simulink library "sm_linear_actuator_lib"  (R2021b)
settings: Solver=ode45  StartTime=0.0  StopTime=10.0  RelTol=1e-3  EnableMultiTasking=on
undefined symbols (not defined in the file or in its folder): X, Y, Z
libraries: sm_lib x28, $bdroot x7
settings Model: Creator=The MathWorks, Inc.  LastModifiedBy=The MathWorks, Inc.
settings SolverCC: AlgebraicLoopSolver=TrustRegion
settings DataIOCC: LimitDataPoints=on  SaveFormat=Array  ReturnWorkspaceOutputs=off
settings OptimizationCC: LifeSpan=inf
settings DebuggingCC: SolverPrmCheckMsg=warning  AllowSymbolicDim=off  SFUnexpectedBacktrackingDiag=warning  SFNoUnconditionalDefaultTransitionDiag=warning  SFExecutionAtInitializationDiag=none  SFMachineParentedDataDiag=warning  ArithmeticOperatorsInVariantConditions=warning
settings HardwareCC: ProdBitPerPointer=32  ProdBitPerSizeT=32  ProdBitPerPtrDiffT=32  ProdLargestAtomicFloat=None  ProdIntDivRoundTo=Undefined  ProdEndianess=Unspecified  ProdWordSize=32  ProdHWDeviceType=32-bit Generic
settings ModelReferenceCC: PropagateSignalLabelsOutOfModel=off
settings SFSimCC: SimUseLocalCustomCode=off  CustomCodeUndefinedFunction=UseInterfaceOnly
settings RTWCC: RTWUseLocalCustomCode=off
settings CodeAppCC: StateflowObjectComments=on
settings GRTTargetCC: TargetLangStandard=C89/C90 (ANSI)
settings ConfigComp: CovMetricSettings=dw  CovSaveCumulativeToWorkspaceVar=on  CovSaveSingleToWorkspaceVar=on  CovExternalEMLEnable=off  CovSFcnEnable=off

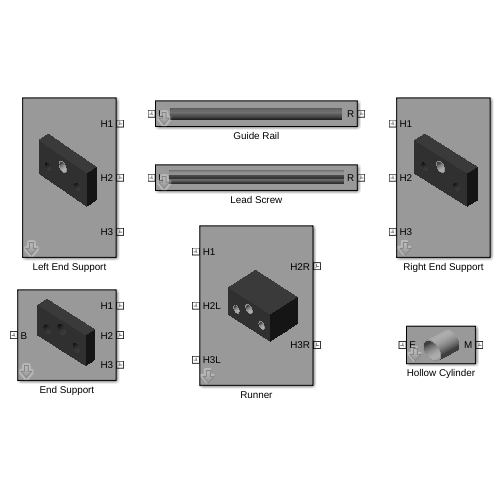
[thumbnail: Simulink's stored preview of the top-level diagram]
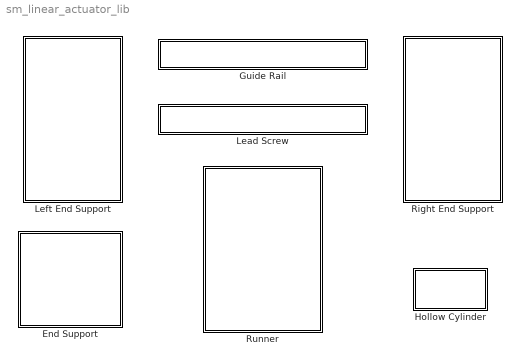
== system sm_linear_actuator_lib ==
  End Support : Subsystem  StatePerturbationForJacobian=1.0e-05  mask(End Support){H=50, W=100, D=20, R1=8.5, R2=7.5, hole1_offset=[0 35], hole2_offset=[30 20], hole3_offset=[-30 20], rho=7800, color=[0.3 0.3 0.3]}
      mask prompts: H "Height (mm)"; W "Width (mm)"; D "Depth (mm)"; R1 "Hole 1 Radius (mm)"; R2 "Holes 2 and 3 Radii (mm)"; hole1_offset "Hole 1 Offset [x y] (mm)"; hole2_offset "Hole 2 Offset [x y] (mm)"; hole3_offset "Hole 3 Offset [x y] (mm)"; rho "Density (kg/m^3)"; color "Color [r g b]"
      mask help:
      | This block models the base part of the end supports for the linear actuator.
      |
      | Port B corresponds to the center of the bottom face of the element.
      |
      | Ports H1, H2 and H3 correspond to the central point of each hole respectively.
      |
      | Each port is located at the midsection of the element.
      mask init:
      | hole_points = 40;
      | 
      | qHole1 = linspace(pi/2, pi/2-2*pi, hole_points);
      | hole1 = [R1*cos(qHole1);
      |          R1*sin(qHole1)+hole1_offset(2)]';
      | 
      | qHole2 = linspace(0, -2*pi, hole_points);
      | hole2 = [R2*cos(qHole2)+hole2_offset(1); 
      |          R2*sin(qHole2)+hole2_offset(2)]';
      | 
      | qHole3 = linspace(pi, -pi, hole_points);
      | hole3 = [R2*cos(qHole3)+hole3_offset(1); 
      |          R2*sin(qHole3)+hole3_offset(2)]';
      | 
      | extrusion_points = [ 0     0;
      |                      0.5*W 0;
      |                      0.5*W hole2_offset(2);
      |                      hole2;
      |                      0.5*W hole2_offset(2);
      |                      0.5*W H;
      |                      0     H;
      |                      hole1;
      |                      0     H;
      |                     -0.5*W H;
      |                     -0.5*W hole3_offset(2);
      |                      hole3;
      |                     -0.5*W hole3_offset(2);
      |                     -0.5*W 0];
      mask DialogControl Container4 Prompt: Dimensions
      mask DialogControl Container9 Prompt: Material Properties
      mask Display:
      | image(fullfile(matlabroot,'toolbox','physmod','sm','smdemos','linear_actuator','images','sm_linear_actuator_end_support.png'));
      | port_label('lconn',1,'B');
      | port_label('rconn',1,'H1');
      | port_label('rconn',2,'H2');
      | port_label('rconn',3,'H3');
  Guide Rail : Subsystem  StatePerturbationForJacobian=1.0e-05  mask(Guide Rail){L=500, R=6, rho=7800, color=[0.5 0.5 0.5]}
      mask prompts: L "Length (mm)"; R "Radius (mm)"; rho "Density (kg/m^3)"; color "Color [r g b]"
      mask help:
      | This block models a guide rail of the linear actuator.
      |
      | The ports L and R correspond to the central points of the two end faces.
      mask DialogControl Container4 Prompt: Dimensions
      mask DialogControl Container5 Prompt: Material Properties
      mask Display:
      | image(fullfile(matlabroot,'toolbox','physmod','sm','smdemos','linear_actuator','images','sm_linear_actuator_guide_rail.png'));
      | port_label('lconn',1,'L');
      | port_label('rconn',1,'R');
  Hollow Cylinder : Subsystem  StatePerturbationForJacobian=1.0e-05  mask(Hollow Cylinder){R=10, T=1, L=20, rho=7800, color=[0.9 0.9 0.9]}
      mask prompts: R "Outer Radius (mm)"; T "Thickness (mm)"; L "Length (mm)"; rho "Density (kg/m^3)"; color "Color [r g b]"
      mask help:
      | This block models a hollow cylinder element.
      |
      | The port E corresponds to the center of the cross-section at the left end.
      |
      | The port M corresponds to the center of the cross-section at the midpoint of the element.
      mask init:
      | iR = R - T;
      | 
      | revolution_points = [iR  L/2;
      |                      iR -L/2;
      |                      R  -L/2;
      |                      R   L/2];
      mask DialogControl Tab01 Prompt: Dimensions
      mask DialogControl Tab02 Prompt: Material Properties
      mask Display:
      | image(fullfile(matlabroot,'toolbox','physmod','sm','smdemos','linear_actuator','images','sm_linear_actuator_hollow_cylinder.png'));
      | port_label('lconn',1,'E');
      | port_label('rconn',1,'M');
  Lead Screw : Subsystem  StatePerturbationForJacobian=1.0e-05  mask(Lead Screw){L=500, R=6, rho=7800, iColor=[0.3 0.3 0.3], oColor=[0.7 0.7 0.7]}
      mask prompts: L "Length (mm)"; R "Radius (mm)"; rho "Density (kg/m^3)"; iColor "Inner Color [r g b]"; oColor "Outer Color [r g b]"
      mask help:
      | This block models the lead screw of the linear actuator.
      |
      | Ports L and R correspond to the central points of the two end faces.
      mask init:
      | x = 0.25*R;
      | 
      | theta = acos(x / R);
      | 
      | theta_arc = pi - 2 * theta;
      | 
      | theta_top_arc = linspace(theta, theta + theta_arc, 20);
      | theta_left_arc = linspace(theta + theta_arc, theta + pi, 20);
      | theta_bottom_arc = linspace(theta + pi, theta + pi + theta_arc, 20);
      | theta_right_arc = linspace(theta + pi + theta_arc, theta + 2*pi, 20);
      | 
      | left_section = [R*cos(theta_left_arc);
      |                   R*sin(theta_left_arc)]';
      | 
      | middle_section = [R*cos(theta_top_arc) R*cos(theta_bottom_arc);
      |                   R*sin(theta_top_arc) R*sin(theta_bottom_arc)]';
      | 
      | right_section = [R*cos(theta_right_arc);
      |                   R*sin(theta_right_arc)]';
      mask DialogControl Container4 Prompt: Dimensions
      mask DialogControl Container5 Prompt: Material Properties
      mask Display:
      | image(fullfile(matlabroot,'toolbox','physmod','sm','smdemos','linear_actuator','images','sm_linear_actuator_lead_screw.png'));
      | port_label('lconn',1,'L');
      | port_label('rconn',1,'R');
  Left End Support : Subsystem  StatePerturbationForJacobian=1.0e-05  mask(Left End Support){H=50, W=100, D=20, R1=7, R2=6, T=1.5, hole1_offset=[0 35], hole2_offset=[30 20], hole3_offset=[-30 20], rho=7800, sColor=[0.3 0.3 0.3], bColor=[0.9 0.9 0.9]}
      mask prompts: H "Height (mm)"; W "Width (mm)"; D "Depth (mm)"; R1 "Hole 1 Radius (mm)"; R2 "Holes 2 and 3 Radii (mm)"; T "Bearing Thickness (mm)"; hole1_offset "Hole 1 Offset [x y] (mm)"; hole2_offset "Hole 2 Offset [x y] (mm)"; hole3_offset "Hole 3 Offset [x y] (mm)"; rho "Density (mg/m^3)"; sColor "Support Color [r g b]"; bColor "Bearing Color [r g b]"
      mask help:
      | This block models the left end support of the linear actuator. The block comprises one End Support and one Hollow Cylinder which models the bearing on which the lead screw rotates.
      |
      | Ports H1, H2 and H3 correspond to the center point of each hole. Each is located on the rear face of the element.
      mask DialogControl Container4 Prompt: Dimensions
      mask DialogControl Container5 Prompt: Material Properties
      mask Display:
      | image(fullfile(matlabroot,'toolbox','physmod','sm','smdemos','linear_actuator','images','sm_linear_actuator_left_end_support.png'));
      | port_label('rconn',1,'H1');
      | port_label('rconn',2,'H2');
      | port_label('rconn',3,'H3');
  Right End Support : Subsystem  StatePerturbationForJacobian=1.0e-05  mask{H=50, W=100, D=20, R1=7, R2=6, T=1.5, hole1_offset=[0 35], hole2_offset=[30 20], hole3_offset=[-30 20], rho=7800, sColor=[0.3 0.3 0.3], bColor=[0.9 0.9 0.9]}
      mask prompts: H "Height (mm)"; W "Width (mm)"; D "Depth (mm)"; R1 "Hole 1 Radius (mm)"; R2 "Holes 2 and 3 Radii (mm)"; T "Bearing Thickness (mm)"; hole1_offset "Hole 1 Offset [x y] (mm)"; hole2_offset "Hole 2 Offset [x y] (mm)"; hole3_offset "Hole 3 Offset [x y] (mm)"; rho "Density (mg/m^3)"; sColor "Support Color [r g b]"; bColor "Bearing Color [r g b]"
      mask help:
      | This block models the right end support of the linear actuator. The block comprises one End Support and one Hollow Cylinder which models the bearing on which the lead screw rotates.
      |
      | Ports H1, H2 and H3 correspond to the center point of each hole. Each is located on the rear face of the element.
      mask DialogControl Container4 Prompt: Dimensions
      mask DialogControl Container5 Prompt: Material Properties
      mask Display:
      | image(fullfile(matlabroot,'toolbox','physmod','sm','smdemos','linear_actuator','images','sm_linear_actuator_right_end_support.png'));
      | port_label('lconn',1,'H1');
      | port_label('lconn',2,'H2');
      | port_label('lconn',3,'H3');
  Runner : Subsystem  StatePerturbationForJacobian=1.0e-05  mask(Runner){H=50, W=100, D=65, R1=7, R2=6, T=1.5, hole1_offset=[0 35], hole2_offset=[30 20], hole3_offset=[-30 20], rho=7800, rColor=[0.3 0.3 0.3], bColor=[0.9 0.9 0.9]}
      mask prompts: H "Height (mm)"; W "Width (mm)"; D "Depth (mm)"; R1 "Hole 1 Radius (mm)"; R2 "Holes 2 and 3 Radii (mm)"; T "Bearing Thickness"; hole1_offset "Hole 1 Offset [x y] (mm)"; hole2_offset "Hole 2 Offset [x y] (mm)"; hole3_offset "Hole 3 Offset [x y] (mm)"; rho "Density (kg/m^3)"; rColor "Runner Color [r g b]"; bColor "Bearing Color [r g b]"
      mask help:
      | This block models the runner of the linear actuator. The block contains three Hollow Cylinder elements which model the bearings on which the runner slides and connect the runner to the lead screw.
      |
      | Port H1 corresponds to the lead screw connection and is located at the central point of hole 1.
      |
      | Ports H2L, H3L, H2R and H3R correspond to the connection points to the guide rails and are located at the center points of the holes on the front and rear faces.
      mask init:
      | hole_points = 40;
      | 
      | qHole1 = linspace(pi/2, pi/2-2*pi, hole_points);
      | r1 = R1+T;
      | hole1 = [r1*cos(qHole1);
      |          r1*sin(qHole1)+hole1_offset(2)]';
      | 
      | qHole2 = linspace(0, -2*pi, hole_points);
      | r2 = R2+T;
      | hole2 = [r2*cos(qHole2)+hole2_offset(1); 
      |          r2*sin(qHole2)+hole2_offset(2)]';
      | 
      | qHole3 = linspace(pi, -pi, hole_points);
      | hole3 = [r2*cos(qHole3)+hole3_offset(1); 
      |          r2*sin(qHole3)+hole3_offset(2)]';
      | 
      | extrusion_points = [ 0     0;
      |                      0.5*W 0;
      |                      0.5*W hole2_offset(2);
      |                      hole2;
      |                      0.5*W hole2_offset(2);
      |                      0.5*W H;
      |                      0     H;
      |                      hole1;
      |                      0     H;
      |                     -0.5*W H;
      |                     -0.5*W hole3_offset(2);
      |                      hole3;
      |                     -0.5*W hole3_offset(2);
      |                     -0.5*W 0];
      mask DialogControl Container4 Prompt: Runner Dimensions
      mask DialogControl Container9 Prompt: Material Properties
      mask Display:
      | image(fullfile(matlabroot,'toolbox','physmod','sm','smdemos','linear_actuator','images','sm_linear_actuator_runner.png'));
      | port_label('lconn',1,'H1');
      | port_label('lconn',2,'H2L');
      | port_label('lconn',3,'H3L');
      | port_label('rconn',1,'H2R');
      | port_label('rconn',2,'H3R');

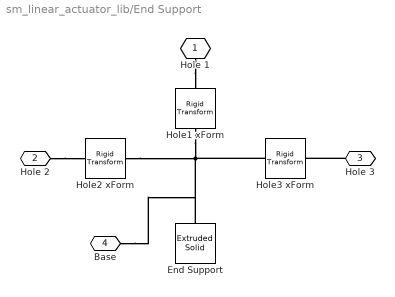
== system sm_linear_actuator_lib/End Support ==
  End Support : sm_lib/Body Elements/Extruded Solid  StatePerturbationForJacobian=1.0e-05  GraphicAmbientColor=[0.15 0.15 0.15 1.0]  BasedOnType=Density  CenterOfMass=[0 0 0]  CenterOfMassUnits=m  GraphicDiffuseColor=color  ExportConvexHullGeometry=off  ExtrusionCrossSection=extrusion_points  ExtrusionCrossSectionUnits=mm  Density=rho  DensityUnits=kg/(m^3)  DoExposeReferenceFrame=on  GraphicEmissiveColor=[0.0 0.0 0.0 1.0]  ExportEntireGeometry=off  ExtrusionLength=D  ExtrusionLengthUnits=mm  ExtrusionType=General  SerializedFrames=<Frames/>  MarkerShape=Sphere  MarkerSize=10  GraphicType=FromGeometry  InertiaType=CalculateFromGeometry  Mass=1  MassUnits=kg  MomentsOfInertia=[1 1 1]  MomentsOfInertiaUnits=kg*m^2  PolygonNumSides=3  GraphicOpacity=1.0  PolygonOuterRadius=1  PolygonOuterRadiusUnits=m  ProductsOfInertia=[0 0 0]  ProductsOfInertiaUnits=kg*m^2  GraphicShininess=75  GraphicSpecularColor=[0.5 0.5 0.5 1.0]  GraphicVisPropType=SimpleVisualProperties
  Hole1 xForm : sm_lib/Frames and Transforms/Rigid Transform  StatePerturbationForJacobian=1.0e-05  TranslationMethod=Cartesian  TranslationStandardOffset=0  TranslationLengthUnit=mm  TranslationStandardAxis=+Z  TranslationCartesianOffset=[hole1_offset 0]  TranslationROffset=0  TranslationROffsetUnits=m  TranslationZOffset=0  TranslationZOffsetUnits=m  TranslationThetaOffset=0  TranslationThetaOffsetUnits=deg  RotationMethod=None  RotationAngleUnits=deg  RotationStandardAxis=+Z  RotationAngle=0.0  RotationArbitraryAxis=[0 0 1]  FollAlignAxisA=+X  BaseAlignAxisA=+Y  FollAlignAxisB=+Y  BaseAlignAxisB=+Z  RotationSequenceAxes=FollowerAxes  RotationSequence=XYX  RotationSequenceAngles=[0 0 0]  RotationSequenceAnglesUnits=deg  RotationMatrix=[1 0 0; 0 1 0; 0 0 1]
  Hole2 xForm : sm_lib/Frames and Transforms/Rigid Transform  StatePerturbationForJacobian=1.0e-05  TranslationMethod=Cartesian  TranslationStandardOffset=0  TranslationLengthUnit=mm  TranslationStandardAxis=+Z  TranslationCartesianOffset=[hole2_offset 0]  TranslationROffset=0  TranslationROffsetUnits=m  TranslationZOffset=0  TranslationZOffsetUnits=m  TranslationThetaOffset=0  TranslationThetaOffsetUnits=deg  RotationMethod=None  RotationAngleUnits=deg  RotationStandardAxis=+Z  RotationAngle=0.0  RotationArbitraryAxis=[0 0 1]  FollAlignAxisA=+X  BaseAlignAxisA=+Y  FollAlignAxisB=+Y  BaseAlignAxisB=+Z  RotationSequenceAxes=FollowerAxes  RotationSequence=XYX  RotationSequenceAngles=[0 0 0]  RotationSequenceAnglesUnits=deg  RotationMatrix=[1 0 0; 0 1 0; 0 0 1]
  Hole3 xForm : sm_lib/Frames and Transforms/Rigid Transform  StatePerturbationForJacobian=1.0e-05  TranslationMethod=Cartesian  TranslationStandardOffset=0  TranslationLengthUnit=mm  TranslationStandardAxis=+Z  TranslationCartesianOffset=[hole3_offset 0]  TranslationROffset=0  TranslationROffsetUnits=m  TranslationZOffset=0  TranslationZOffsetUnits=m  TranslationThetaOffset=0  TranslationThetaOffsetUnits=deg  RotationMethod=None  RotationAngleUnits=deg  RotationStandardAxis=+Z  RotationAngle=0.0  RotationArbitraryAxis=[0 0 1]  FollAlignAxisA=+X  BaseAlignAxisA=+Y  FollAlignAxisB=+Y  BaseAlignAxisB=+Z  RotationSequenceAxes=FollowerAxes  RotationSequence=XYX  RotationSequenceAngles=[0 0 0]  RotationSequenceAnglesUnits=deg  RotationMatrix=[1 0 0; 0 1 0; 0 0 1]
  Hole 1 : PMIOPort  StatePerturbationForJacobian=1.0e-05  Side=Right
  Hole 2 : PMIOPort  StatePerturbationForJacobian=1.0e-05  Port=2  Side=Right
  Hole 3 : PMIOPort  StatePerturbationForJacobian=1.0e-05  Port=3  Side=Right
  Base : PMIOPort  StatePerturbationForJacobian=1.0e-05  Port=4  Side=Left
  connections:
  Hole 3/RConn1 -- Hole3 xForm/RConn1
  Hole 2/RConn1 -- Hole2 xForm/RConn1
  Hole 1/RConn1 -- Hole1 xForm/RConn1
  Hole3 xForm/LConn1 -- Base/RConn1 -- End Support/RConn1 -- Hole2 xForm/LConn1 -- Hole1 xForm/LConn1

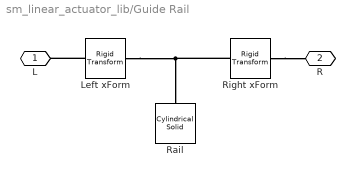
== system sm_linear_actuator_lib/Guide Rail ==
  Left xForm : sm_lib/Frames and Transforms/Rigid Transform  StatePerturbationForJacobian=1.0e-05  TranslationMethod=StandardAxis  TranslationStandardOffset=L/2  TranslationLengthUnit=mm  TranslationStandardAxis=+Z  TranslationCartesianOffset=[0 0 0]  TranslationROffset=0  TranslationROffsetUnits=m  TranslationZOffset=0  TranslationZOffsetUnits=m  TranslationThetaOffset=0  TranslationThetaOffsetUnits=deg  RotationMethod=AlignedAxes  RotationAngleUnits=deg  RotationStandardAxis=+Z  RotationAngle=0.0  RotationArbitraryAxis=[0 0 1]  FollAlignAxisA=+Z  BaseAlignAxisA=-Z  FollAlignAxisB=+Y  BaseAlignAxisB=+Y  RotationSequenceAxes=FollowerAxes  RotationSequence=XYX  RotationSequenceAngles=[0 0 0]  RotationSequenceAnglesUnits=deg  RotationMatrix=[1 0 0; 0 1 0; 0 0 1]
  Rail : sm_lib/Body Elements/Cylindrical Solid  StatePerturbationForJacobian=1.0e-05  GraphicAmbientColor=[0.15 0.15 0.15 1.0]  BasedOnType=Density  CenterOfMass=[0 0 0]  CenterOfMassUnits=m  GraphicDiffuseColor=color  CylinderLength=L  CylinderLengthUnits=mm  CylinderRadius=R  CylinderRadiusUnits=mm  Density=rho  DensityUnits=kg/(m^3)  DoExposeReferenceFrame=on  GraphicEmissiveColor=[0.0 0.0 0.0 1.0]  ExportEntireGeometry=off  SerializedFrames=<Frames/>  MarkerShape=Sphere  MarkerSize=10  GraphicType=FromGeometry  InertiaType=CalculateFromGeometry  Mass=1  MassUnits=kg  MomentsOfInertia=[1 1 1]  MomentsOfInertiaUnits=kg*m^2  GraphicOpacity=1.0  ProductsOfInertia=[0 0 0]  ProductsOfInertiaUnits=kg*m^2  GraphicShininess=75  GraphicSpecularColor=[0.5 0.5 0.5 1.0]  GraphicVisPropType=SimpleVisualProperties
  Right xForm : sm_lib/Frames and Transforms/Rigid Transform  StatePerturbationForJacobian=1.0e-05  TranslationMethod=StandardAxis  TranslationStandardOffset=L/2  TranslationLengthUnit=mm  TranslationStandardAxis=-Z  TranslationCartesianOffset=[0 0 0]  TranslationROffset=0  TranslationROffsetUnits=m  TranslationZOffset=0  TranslationZOffsetUnits=m  TranslationThetaOffset=0  TranslationThetaOffsetUnits=deg  RotationMethod=None  RotationAngleUnits=deg  RotationStandardAxis=+Z  RotationAngle=0.0  RotationArbitraryAxis=[0 0 1]  FollAlignAxisA=+Z  BaseAlignAxisA=+Z  FollAlignAxisB=+Y  BaseAlignAxisB=+Y  RotationSequenceAxes=FollowerAxes  RotationSequence=XYX  RotationSequenceAngles=[0 0 0]  RotationSequenceAnglesUnits=deg  RotationMatrix=[1 0 0; 0 1 0; 0 0 1]
  L : PMIOPort  StatePerturbationForJacobian=1.0e-05  Side=Left
  R : PMIOPort  StatePerturbationForJacobian=1.0e-05  Port=2  Side=Right
  connections:
  Left xForm/RConn1 -- L/RConn1
  Right xForm/RConn1 -- R/RConn1
  Left xForm/LConn1 -- Rail/RConn1 -- Right xForm/LConn1

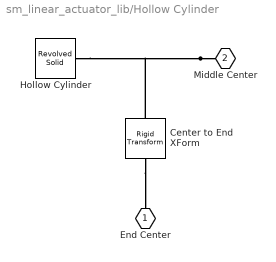
== system sm_linear_actuator_lib/Hollow Cylinder ==
  Center to End XForm : sm_lib/Frames and Transforms/Rigid Transform  StatePerturbationForJacobian=1.0e-05  TranslationMethod=StandardAxis  TranslationStandardOffset=L/2  TranslationLengthUnit=mm  TranslationStandardAxis=-Z  TranslationCartesianOffset=[0 0 0]  TranslationROffset=0  TranslationROffsetUnits=m  TranslationZOffset=0  TranslationZOffsetUnits=m  TranslationThetaOffset=0  TranslationThetaOffsetUnits=deg  RotationMethod=None  RotationAngleUnits=deg  RotationStandardAxis=+Z  RotationAngle=0  RotationArbitraryAxis=[0 0 1]  FollAlignAxisA=+X  BaseAlignAxisA=+Y  FollAlignAxisB=+Y  BaseAlignAxisB=+Z  RotationSequenceAxes=FollowerAxes  RotationSequence=XYX  RotationSequenceAngles=[0 0 0]  RotationSequenceAnglesUnits=deg  RotationMatrix=[1 0 0; 0 1 0; 0 0 1]
  Hollow Cylinder : sm_lib/Body Elements/Revolved Solid  StatePerturbationForJacobian=1.0e-05  GraphicAmbientColor=[0.15 0.15 0.15 1.0]  BasedOnType=Density  CenterOfMass=[0 0 0]  CenterOfMassUnits=m  GraphicDiffuseColor=color  ExportConvexHullGeometry=off  Density=rho  DensityUnits=kg/(m^3)  DoExposeReferenceFrame=on  GraphicEmissiveColor=[0.0 0.0 0.0 1.0]  ExportEntireGeometry=off  SerializedFrames=<Frames/>  MarkerShape=Sphere  MarkerSize=10  GraphicType=FromGeometry  InertiaType=CalculateFromGeometry  Mass=1  MassUnits=kg  MomentsOfInertia=[1 1 1]  MomentsOfInertiaUnits=kg*m^2  GraphicOpacity=1.0  ProductsOfInertia=[0 0 0]  ProductsOfInertiaUnits=kg*m^2  RevolutionCrossSection=revolution_points  RevolutionCrossSectionUnits=mm  RevolutionAngle=180  RevolutionAngleUnits=deg  RevolutionExtent=Full  GraphicShininess=75  GraphicSpecularColor=[0.5 0.5 0.5 1.0]  GraphicVisPropType=SimpleVisualProperties
  End Center : PMIOPort  StatePerturbationForJacobian=1.0e-05  Side=Left
  Middle Center : PMIOPort  StatePerturbationForJacobian=1.0e-05  Port=2  Side=Right
  connections:
  Center to End XForm/RConn1 -- End Center/RConn1
  Middle Center/RConn1 -- Center to End XForm/LConn1 -- Hollow Cylinder/RConn1

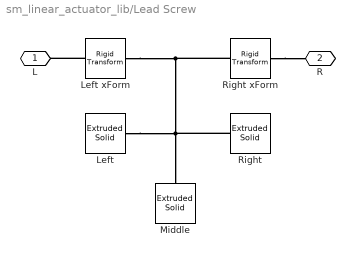
== system sm_linear_actuator_lib/Lead Screw ==
  Left : sm_lib/Body Elements/Extruded Solid  StatePerturbationForJacobian=1.0e-05  GraphicAmbientColor=[0.15 0.15 0.15 1.0]  BasedOnType=Density  CenterOfMass=[0 0 0]  CenterOfMassUnits=m  GraphicDiffuseColor=oColor  ExportConvexHullGeometry=off  ExtrusionCrossSection=left_section  ExtrusionCrossSectionUnits=mm  Density=rho  DensityUnits=kg/(m^3)  DoExposeReferenceFrame=on  GraphicEmissiveColor=[0.0 0.0 0.0 1.0]  ExportEntireGeometry=off  ExtrusionLength=L  ExtrusionLengthUnits=mm  ExtrusionType=General  SerializedFrames=<Frames/>  MarkerShape=Sphere  MarkerSize=10  GraphicType=FromGeometry  InertiaType=CalculateFromGeometry  Mass=1  MassUnits=kg  MomentsOfInertia=[1 1 1]  MomentsOfInertiaUnits=kg*m^2  PolygonNumSides=3  GraphicOpacity=1.0  PolygonOuterRadius=1  PolygonOuterRadiusUnits=m  ProductsOfInertia=[0 0 0]  ProductsOfInertiaUnits=kg*m^2  GraphicShininess=75  GraphicSpecularColor=[0.5 0.5 0.5 1.0]  GraphicVisPropType=SimpleVisualProperties
  Left xForm : sm_lib/Frames and Transforms/Rigid Transform  StatePerturbationForJacobian=1.0e-05  TranslationMethod=StandardAxis  TranslationStandardOffset=L/2  TranslationLengthUnit=mm  TranslationStandardAxis=+Z  TranslationCartesianOffset=[0 0 0]  TranslationROffset=0  TranslationROffsetUnits=m  TranslationZOffset=0  TranslationZOffsetUnits=m  TranslationThetaOffset=0  TranslationThetaOffsetUnits=deg  RotationMethod=AlignedAxes  RotationAngleUnits=deg  RotationStandardAxis=+Z  RotationAngle=0.0  RotationArbitraryAxis=[0 0 1]  FollAlignAxisA=+Z  BaseAlignAxisA=-Z  FollAlignAxisB=+Y  BaseAlignAxisB=+Y  RotationSequenceAxes=FollowerAxes  RotationSequence=XYX  RotationSequenceAngles=[0 0 0]  RotationSequenceAnglesUnits=deg  RotationMatrix=[1 0 0; 0 1 0; 0 0 1]
  Middle : sm_lib/Body Elements/Extruded Solid  StatePerturbationForJacobian=1.0e-05  GraphicAmbientColor=[0.15 0.15 0.15 1.0]  BasedOnType=Density  CenterOfMass=[0 0 0]  CenterOfMassUnits=m  GraphicDiffuseColor=iColor  ExportConvexHullGeometry=off  ExtrusionCrossSection=middle_section  ExtrusionCrossSectionUnits=mm  Density=rho  DensityUnits=kg/(m^3)  DoExposeReferenceFrame=on  GraphicEmissiveColor=[0.0 0.0 0.0 1.0]  ExportEntireGeometry=off  ExtrusionLength=L  ExtrusionLengthUnits=mm  ExtrusionType=General  SerializedFrames=<Frames/>  MarkerShape=Sphere  MarkerSize=10  GraphicType=FromGeometry  InertiaType=CalculateFromGeometry  Mass=1  MassUnits=kg  MomentsOfInertia=[1 1 1]  MomentsOfInertiaUnits=kg*m^2  PolygonNumSides=3  GraphicOpacity=1.0  PolygonOuterRadius=1  PolygonOuterRadiusUnits=m  ProductsOfInertia=[0 0 0]  ProductsOfInertiaUnits=kg*m^2  GraphicShininess=75  GraphicSpecularColor=[0.5 0.5 0.5 1.0]  GraphicVisPropType=SimpleVisualProperties
  Right : sm_lib/Body Elements/Extruded Solid  StatePerturbationForJacobian=1.0e-05  GraphicAmbientColor=[0.15 0.15 0.15 1.0]  BasedOnType=Density  CenterOfMass=[0 0 0]  CenterOfMassUnits=m  GraphicDiffuseColor=oColor  ExportConvexHullGeometry=off  ExtrusionCrossSection=right_section  ExtrusionCrossSectionUnits=mm  Density=rho  DensityUnits=kg/(m^3)  DoExposeReferenceFrame=on  GraphicEmissiveColor=[0.0 0.0 0.0 1.0]  ExportEntireGeometry=off  ExtrusionLength=L  ExtrusionLengthUnits=mm  ExtrusionType=General  SerializedFrames=<Frames/>  MarkerShape=Sphere  MarkerSize=10  GraphicType=FromGeometry  InertiaType=CalculateFromGeometry  Mass=1  MassUnits=kg  MomentsOfInertia=[1 1 1]  MomentsOfInertiaUnits=kg*m^2  PolygonNumSides=3  GraphicOpacity=1.0  PolygonOuterRadius=1  PolygonOuterRadiusUnits=m  ProductsOfInertia=[0 0 0]  ProductsOfInertiaUnits=kg*m^2  GraphicShininess=75  GraphicSpecularColor=[0.5 0.5 0.5 1.0]  GraphicVisPropType=SimpleVisualProperties
  Right xForm : sm_lib/Frames and Transforms/Rigid Transform  StatePerturbationForJacobian=1.0e-05  TranslationMethod=StandardAxis  TranslationStandardOffset=L/2  TranslationLengthUnit=mm  TranslationStandardAxis=-Z  TranslationCartesianOffset=[0 0 0]  TranslationROffset=0  TranslationROffsetUnits=m  TranslationZOffset=0  TranslationZOffsetUnits=m  TranslationThetaOffset=0  TranslationThetaOffsetUnits=deg  RotationMethod=None  RotationAngleUnits=deg  RotationStandardAxis=+Z  RotationAngle=0.0  RotationArbitraryAxis=[0 0 1]  FollAlignAxisA=+Z  BaseAlignAxisA=+Z  FollAlignAxisB=+Y  BaseAlignAxisB=+Y  RotationSequenceAxes=FollowerAxes  RotationSequence=XYX  RotationSequenceAngles=[0 0 0]  RotationSequenceAnglesUnits=deg  RotationMatrix=[1 0 0; 0 1 0; 0 0 1]
  L : PMIOPort  StatePerturbationForJacobian=1.0e-05  Side=Left
  R : PMIOPort  StatePerturbationForJacobian=1.0e-05  Port=2  Side=Right
  connections:
  Right xForm/LConn1 -- Right/RConn1 -- Left/RConn1 -- Middle/RConn1 -- Left xForm/LConn1
  Right xForm/RConn1 -- R/RConn1
  Left xForm/RConn1 -- L/RConn1

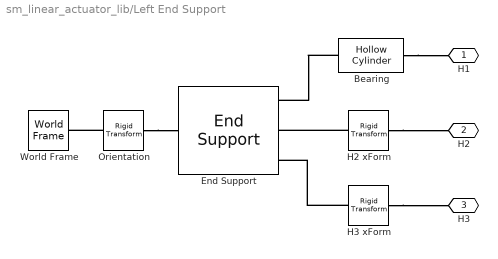
== system sm_linear_actuator_lib/Left End Support ==
  Bearing : $bdroot/Hollow Cylinder  StatePerturbationForJacobian=1.0e-05  R=R1+T  T=T  L=D  rho=rho  color=bColor
  End Support : $bdroot/End Support  StatePerturbationForJacobian=1.0e-05  H=H  W=W  D=D  R1=R1+T  R2=R2  hole1_offset=hole1_offset  hole2_offset=hole2_offset  hole3_offset=hole3_offset  rho=rho  color=sColor
  H2 xForm : sm_lib/Frames and Transforms/Rigid Transform  StatePerturbationForJacobian=1.0e-05  TranslationMethod=StandardAxis  TranslationStandardOffset=D/2  TranslationLengthUnit=mm  TranslationStandardAxis=-Z  TranslationCartesianOffset=[0 0 0]  TranslationROffset=0  TranslationROffsetUnits=m  TranslationZOffset=0  TranslationZOffsetUnits=m  TranslationThetaOffset=0  TranslationThetaOffsetUnits=deg  RotationMethod=None  RotationAngleUnits=deg  RotationStandardAxis=+Z  RotationAngle=0.0  RotationArbitraryAxis=[0 0 1]  FollAlignAxisA=+X  BaseAlignAxisA=+Y  FollAlignAxisB=+Y  BaseAlignAxisB=+Z  RotationSequenceAxes=FollowerAxes  RotationSequence=XYX  RotationSequenceAngles=[0 0 0]  RotationSequenceAnglesUnits=deg  RotationMatrix=[1 0 0; 0 1 0; 0 0 1]
  H3 xForm : sm_lib/Frames and Transforms/Rigid Transform  StatePerturbationForJacobian=1.0e-05  TranslationMethod=StandardAxis  TranslationStandardOffset=D/2  TranslationLengthUnit=mm  TranslationStandardAxis=-Z  TranslationCartesianOffset=[0 0 0]  TranslationROffset=0  TranslationROffsetUnits=m  TranslationZOffset=0  TranslationZOffsetUnits=m  TranslationThetaOffset=0  TranslationThetaOffsetUnits=deg  RotationMethod=None  RotationAngleUnits=deg  RotationStandardAxis=+Z  RotationAngle=0.0  RotationArbitraryAxis=[0 0 1]  FollAlignAxisA=+X  BaseAlignAxisA=+Y  FollAlignAxisB=+Y  BaseAlignAxisB=+Z  RotationSequenceAxes=FollowerAxes  RotationSequence=XYX  RotationSequenceAngles=[0 0 0]  RotationSequenceAnglesUnits=deg  RotationMatrix=[1 0 0; 0 1 0; 0 0 1]
  Orientation : sm_lib/Frames and Transforms/Rigid Transform  StatePerturbationForJacobian=1.0e-05  TranslationMethod=None  TranslationStandardOffset=0  TranslationLengthUnit=m  TranslationStandardAxis=+Z  TranslationCartesianOffset=[0 0 0]  TranslationROffset=0  TranslationROffsetUnits=m  TranslationZOffset=0  TranslationZOffsetUnits=m  TranslationThetaOffset=0  TranslationThetaOffsetUnits=deg  RotationMethod=AlignedAxes  RotationAngleUnits=deg  RotationStandardAxis=+Z  RotationAngle=0.0  RotationArbitraryAxis=[0 0 1]  FollAlignAxisA=+Z  BaseAlignAxisA=+Y  FollAlignAxisB=+Y  BaseAlignAxisB=+Z  RotationSequenceAxes=FollowerAxes  RotationSequence=XYX  RotationSequenceAngles=[0 0 0]  RotationSequenceAnglesUnits=deg  RotationMatrix=[1 0 0; 0 1 0; 0 0 1]
  World Frame : sm_lib/Frames and Transforms/World Frame  StatePerturbationForJacobian=1.0e-05
  H1 : PMIOPort  StatePerturbationForJacobian=1.0e-05  Side=Right
  H2 : PMIOPort  StatePerturbationForJacobian=1.0e-05  Port=2  Side=Right
  H3 : PMIOPort  StatePerturbationForJacobian=1.0e-05  Port=3  Side=Right
  connections:
  Orientation/RConn1 -- End Support/LConn1
  Bearing/LConn1 -- H1/RConn1
  H3 xForm/LConn1 -- End Support/RConn3
  H3 xForm/RConn1 -- H3/RConn1
  H2 xForm/RConn1 -- H2/RConn1
  H2 xForm/LConn1 -- End Support/RConn2
  Bearing/RConn1 -- End Support/RConn1
  Orientation/LConn1 -- World Frame/RConn1

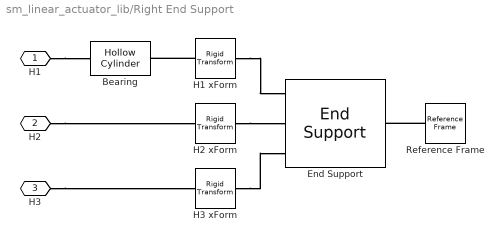
== system sm_linear_actuator_lib/Right End Support ==
  Bearing : $bdroot/Hollow Cylinder  StatePerturbationForJacobian=1.0e-05  R=R1+T  T=T  L=D  rho=rho  color=bColor
  End Support : $bdroot/End Support  StatePerturbationForJacobian=1.0e-05  H=H  W=W  D=D  R1=R1+T  R2=R2  hole1_offset=hole1_offset  hole2_offset=hole2_offset  hole3_offset=hole3_offset  rho=rho  color=sColor
  H1 xForm : sm_lib/Frames and Transforms/Rigid Transform  StatePerturbationForJacobian=1.0e-05  TranslationMethod=None  TranslationStandardOffset=0  TranslationLengthUnit=m  TranslationStandardAxis=+Z  TranslationCartesianOffset=[0 0 0]  TranslationROffset=0  TranslationROffsetUnits=m  TranslationZOffset=0  TranslationZOffsetUnits=m  TranslationThetaOffset=0  TranslationThetaOffsetUnits=deg  RotationMethod=AlignedAxes  RotationAngleUnits=deg  RotationStandardAxis=+Z  RotationAngle=0.0  RotationArbitraryAxis=[0 0 1]  FollAlignAxisA=+Z  BaseAlignAxisA=-Z  FollAlignAxisB=+Y  BaseAlignAxisB=+Y  RotationSequenceAxes=FollowerAxes  RotationSequence=XYX  RotationSequenceAngles=[0 0 0]  RotationSequenceAnglesUnits=deg  RotationMatrix=[1 0 0; 0 1 0; 0 0 1]
  H2 xForm : sm_lib/Frames and Transforms/Rigid Transform  StatePerturbationForJacobian=1.0e-05  TranslationMethod=StandardAxis  TranslationStandardOffset=D/2  TranslationLengthUnit=mm  TranslationStandardAxis=+Z  TranslationCartesianOffset=[0 0 0]  TranslationROffset=0  TranslationROffsetUnits=m  TranslationZOffset=0  TranslationZOffsetUnits=m  TranslationThetaOffset=0  TranslationThetaOffsetUnits=deg  RotationMethod=AlignedAxes  RotationAngleUnits=deg  RotationStandardAxis=+Z  RotationAngle=0.0  RotationArbitraryAxis=[0 0 1]  FollAlignAxisA=+Z  BaseAlignAxisA=-Z  FollAlignAxisB=+Y  BaseAlignAxisB=+Y  RotationSequenceAxes=FollowerAxes  RotationSequence=XYX  RotationSequenceAngles=[0 0 0]  RotationSequenceAnglesUnits=deg  RotationMatrix=[1 0 0; 0 1 0; 0 0 1]
  H3 xForm : sm_lib/Frames and Transforms/Rigid Transform  StatePerturbationForJacobian=1.0e-05  TranslationMethod=StandardAxis  TranslationStandardOffset=D/2  TranslationLengthUnit=mm  TranslationStandardAxis=+Z  TranslationCartesianOffset=[0 0 0]  TranslationROffset=0  TranslationROffsetUnits=m  TranslationZOffset=0  TranslationZOffsetUnits=m  TranslationThetaOffset=0  TranslationThetaOffsetUnits=deg  RotationMethod=AlignedAxes  RotationAngleUnits=deg  RotationStandardAxis=+Z  RotationAngle=0.0  RotationArbitraryAxis=[0 0 1]  FollAlignAxisA=+Z  BaseAlignAxisA=-Z  FollAlignAxisB=+Y  BaseAlignAxisB=+Y  RotationSequenceAxes=FollowerAxes  RotationSequence=XYX  RotationSequenceAngles=[0 0 0]  RotationSequenceAnglesUnits=deg  RotationMatrix=[1 0 0; 0 1 0; 0 0 1]
  Reference Frame : sm_lib/Frames and Transforms/Reference Frame  StatePerturbationForJacobian=1.0e-05
  H1 : PMIOPort  StatePerturbationForJacobian=1.0e-05  Side=Left
  H2 : PMIOPort  StatePerturbationForJacobian=1.0e-05  Port=2  Side=Left
  H3 : PMIOPort  StatePerturbationForJacobian=1.0e-05  Port=3  Side=Left
  connections:
  Reference Frame/RConn1 -- End Support/LConn1
  H3/RConn1 -- H3 xForm/RConn1
  H2/RConn1 -- H2 xForm/RConn1
  H1/RConn1 -- Bearing/LConn1
  H1 xForm/RConn1 -- Bearing/RConn1
  H2 xForm/LConn1 -- End Support/RConn2
  H3 xForm/LConn1 -- End Support/RConn3
  H1 xForm/LConn1 -- End Support/RConn1

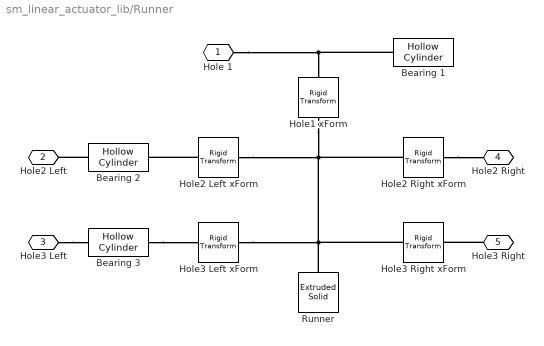
== system sm_linear_actuator_lib/Runner ==
  Bearing 1 : $bdroot/Hollow Cylinder  StatePerturbationForJacobian=1.0e-05  R=R1+T  T=T  L=D  rho=rho  color=bColor
  Bearing 2 : $bdroot/Hollow Cylinder  StatePerturbationForJacobian=1.0e-05  R=R2+T  T=T  L=D  rho=rho  color=bColor
  Bearing 3 : $bdroot/Hollow Cylinder  StatePerturbationForJacobian=1.0e-05  R=R2+T  T=T  L=D  rho=rho  color=bColor
  Hole1 xForm : sm_lib/Frames and Transforms/Rigid Transform  StatePerturbationForJacobian=1.0e-05  TranslationMethod=Cartesian  TranslationStandardOffset=0  TranslationLengthUnit=mm  TranslationStandardAxis=+Z  TranslationCartesianOffset=[hole1_offset 0]  TranslationROffset=0  TranslationROffsetUnits=m  TranslationZOffset=0  TranslationZOffsetUnits=m  TranslationThetaOffset=0  TranslationThetaOffsetUnits=deg  RotationMethod=None  RotationAngleUnits=deg  RotationStandardAxis=+Z  RotationAngle=0.0  RotationArbitraryAxis=[0 0 1]  FollAlignAxisA=+X  BaseAlignAxisA=+Y  FollAlignAxisB=+Y  BaseAlignAxisB=+Z  RotationSequenceAxes=FollowerAxes  RotationSequence=XYX  RotationSequenceAngles=[0 0 0]  RotationSequenceAnglesUnits=deg  RotationMatrix=[1 0 0; 0 1 0; 0 0 1]
  Hole2 Left xForm : sm_lib/Frames and Transforms/Rigid Transform  StatePerturbationForJacobian=1.0e-05  TranslationMethod=Cartesian  TranslationStandardOffset=0  TranslationLengthUnit=mm  TranslationStandardAxis=+Z  TranslationCartesianOffset=[hole2_offset 0]  TranslationROffset=0  TranslationROffsetUnits=m  TranslationZOffset=0  TranslationZOffsetUnits=m  TranslationThetaOffset=0  TranslationThetaOffsetUnits=deg  RotationMethod=None  RotationAngleUnits=deg  RotationStandardAxis=+Z  RotationAngle=0.0  RotationArbitraryAxis=[0 0 1]  FollAlignAxisA=+X  BaseAlignAxisA=+Y  FollAlignAxisB=+Y  BaseAlignAxisB=+Z  RotationSequenceAxes=FollowerAxes  RotationSequence=XYX  RotationSequenceAngles=[0 0 0]  RotationSequenceAnglesUnits=deg  RotationMatrix=[1 0 0; 0 1 0; 0 0 1]
  Hole2 Right xForm : sm_lib/Frames and Transforms/Rigid Transform  StatePerturbationForJacobian=1.0e-05  TranslationMethod=Cartesian  TranslationStandardOffset=0  TranslationLengthUnit=mm  TranslationStandardAxis=+Z  TranslationCartesianOffset=[hole2_offset D/2]  TranslationROffset=0  TranslationROffsetUnits=m  TranslationZOffset=0  TranslationZOffsetUnits=m  TranslationThetaOffset=0  TranslationThetaOffsetUnits=deg  RotationMethod=AlignedAxes  RotationAngleUnits=deg  RotationStandardAxis=+Z  RotationAngle=0.0  RotationArbitraryAxis=[0 0 1]  FollAlignAxisA=+Z  BaseAlignAxisA=-Z  FollAlignAxisB=+Y  BaseAlignAxisB=+Y  RotationSequenceAxes=FollowerAxes  RotationSequence=XYX  RotationSequenceAngles=[0 0 0]  RotationSequenceAnglesUnits=deg  RotationMatrix=[1 0 0; 0 1 0; 0 0 1]
  Hole3 Left xForm : sm_lib/Frames and Transforms/Rigid Transform  StatePerturbationForJacobian=1.0e-05  TranslationMethod=Cartesian  TranslationStandardOffset=0  TranslationLengthUnit=mm  TranslationStandardAxis=+Z  TranslationCartesianOffset=[hole3_offset 0]  TranslationROffset=0  TranslationROffsetUnits=m  TranslationZOffset=0  TranslationZOffsetUnits=m  TranslationThetaOffset=0  TranslationThetaOffsetUnits=deg  RotationMethod=None  RotationAngleUnits=deg  RotationStandardAxis=+Z  RotationAngle=0.0  RotationArbitraryAxis=[0 0 1]  FollAlignAxisA=+X  BaseAlignAxisA=+Y  FollAlignAxisB=+Y  BaseAlignAxisB=+Z  RotationSequenceAxes=FollowerAxes  RotationSequence=XYX  RotationSequenceAngles=[0 0 0]  RotationSequenceAnglesUnits=deg  RotationMatrix=[1 0 0; 0 1 0; 0 0 1]
  Hole3 Right xForm : sm_lib/Frames and Transforms/Rigid Transform  StatePerturbationForJacobian=1.0e-05  TranslationMethod=Cartesian  TranslationStandardOffset=0  TranslationLengthUnit=mm  TranslationStandardAxis=+Z  TranslationCartesianOffset=[hole3_offset D/2]  TranslationROffset=0  TranslationROffsetUnits=m  TranslationZOffset=0  TranslationZOffsetUnits=m  TranslationThetaOffset=0  TranslationThetaOffsetUnits=deg  RotationMethod=AlignedAxes  RotationAngleUnits=deg  RotationStandardAxis=+Z  RotationAngle=0.0  RotationArbitraryAxis=[0 0 1]  FollAlignAxisA=+Z  BaseAlignAxisA=-Z  FollAlignAxisB=+Y  BaseAlignAxisB=+Y  RotationSequenceAxes=FollowerAxes  RotationSequence=XYX  RotationSequenceAngles=[0 0 0]  RotationSequenceAnglesUnits=deg  RotationMatrix=[1 0 0; 0 1 0; 0 0 1]
  Runner : sm_lib/Body Elements/Extruded Solid  StatePerturbationForJacobian=1.0e-05  GraphicAmbientColor=[0.15 0.15 0.15 1.0]  BasedOnType=Density  CenterOfMass=[0 0 0]  CenterOfMassUnits=m  GraphicDiffuseColor=rColor  ExportConvexHullGeometry=off  ExtrusionCrossSection=extrusion_points  ExtrusionCrossSectionUnits=mm  Density=rho  DensityUnits=kg/(m^3)  DoExposeReferenceFrame=on  GraphicEmissiveColor=[0.0 0.0 0.0 1.0]  ExportEntireGeometry=off  ExtrusionLength=D  ExtrusionLengthUnits=mm  ExtrusionType=General  SerializedFrames=<Frames/>  MarkerShape=Sphere  MarkerSize=10  GraphicType=FromGeometry  InertiaType=CalculateFromGeometry  Mass=1  MassUnits=kg  MomentsOfInertia=[1 1 1]  MomentsOfInertiaUnits=kg*m^2  PolygonNumSides=3  GraphicOpacity=1.0  PolygonOuterRadius=1  PolygonOuterRadiusUnits=m  ProductsOfInertia=[0 0 0]  ProductsOfInertiaUnits=kg*m^2  GraphicShininess=75  GraphicSpecularColor=[0.5 0.5 0.5 1.0]  GraphicVisPropType=SimpleVisualProperties
  Hole 1 : PMIOPort  StatePerturbationForJacobian=1.0e-05  Side=Left
  Hole2 Left : PMIOPort  StatePerturbationForJacobian=1.0e-05  Port=2  Side=Left
  Hole3 Left : PMIOPort  StatePerturbationForJacobian=1.0e-05  Port=3  Side=Left
  Hole2 Right : PMIOPort  StatePerturbationForJacobian=1.0e-05  Port=4  Side=Right
  Hole3 Right : PMIOPort  StatePerturbationForJacobian=1.0e-05  Port=5  Side=Right
  connections:
  Runner/RConn1 -- Hole2 Right xForm/LConn1 -- Hole2 Left xForm/LConn1 -- Hole1 xForm/LConn1 -- Hole3 Right xForm/LConn1 -- Hole3 Left xForm/LConn1
  Hole 1/RConn1 -- Hole1 xForm/RConn1 -- Bearing 1/RConn1
  Bearing 2/LConn1 -- Hole2 Left/RConn1
  Hole3 Right/RConn1 -- Hole3 Right xForm/RConn1
  Hole3 Left/RConn1 -- Bearing 3/LConn1
  Hole2 Right xForm/RConn1 -- Hole2 Right/RConn1
  Bearing 3/RConn1 -- Hole3 Left xForm/RConn1
  Hole2 Left xForm/RConn1 -- Bearing 2/RConn1
